simulink model "MovementMaker"  (R2021b)
settings: Solver=FixedStepAuto  StartTime=0.0  StopTime=10.0  FixedStep=.01  RelTol=1e-3
settings Model: Creator=Spino.shop  LastModifiedBy=Spino.shop

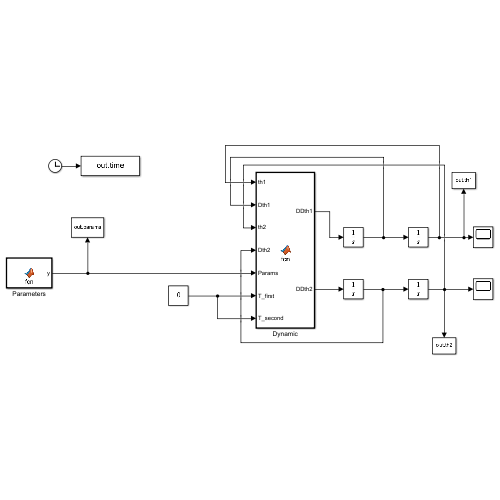
[thumbnail: Simulink's stored preview of the top-level diagram]
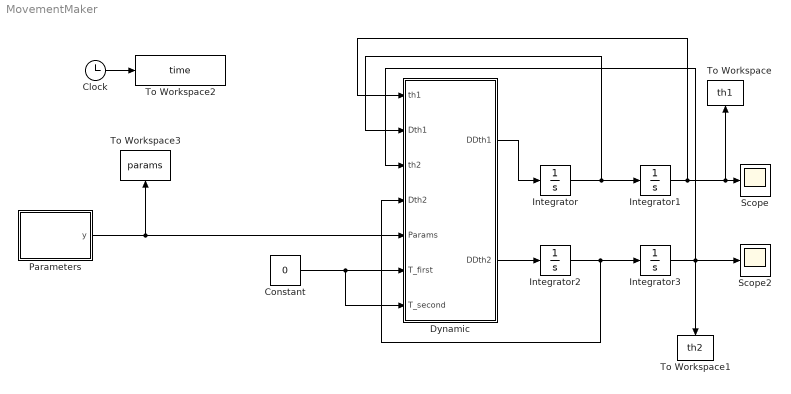
== system MovementMaker ==
  Clock : Clock
  Constant : Constant  Value=0
  Dynamic : MATLAB Function  TreatAsAtomicUnit=on
  Integrator{,1..3} (4 alike) : Integrator
  Parameters : MATLAB Function  TreatAsAtomicUnit=on
  Scope : Scope
  Scope2 : Scope
  To Workspace : ToWorkspace  VariableName=th1  SampleTime=-1
      settings: Save2DSignal=2-D array (concatenate along first dimension)
  To Workspace1 : ToWorkspace  VariableName=th2  SampleTime=-1
      settings: Save2DSignal=2-D array (concatenate along first dimension)
  To Workspace2 : ToWorkspace  VariableName=time  SampleTime=-1
      settings: Save2DSignal=2-D array (concatenate along first dimension)
  To Workspace3 : ToWorkspace  VariableName=params
      settings: MaxDataPoints=1  Save2DSignal=2-D array (concatenate along first dimension)
  wires:
  Integrator/1 -> Dynamic/2(Dth1), Integrator1/1
  Dynamic/1(DDth1) -> Integrator/1
  Parameters/1(y) -> To Workspace3/1, Dynamic/5(Params)
  Clock/1 -> To Workspace2/1
  Integrator2/1 -> Dynamic/4(Dth2), Integrator3/1
  Dynamic/2(DDth2) -> Integrator2/1
  Integrator1/1 -> Dynamic/1(th1), Scope/1, To Workspace/1
  Integrator3/1 -> Dynamic/3(th2), Scope2/1, To Workspace1/1
  Constant/1 -> Dynamic/6(T_first), Dynamic/7(T_second)

== matlab function MovementMaker/Dynamic ==
  data: th1 input; DDth1 output; Dth1 input; th2 input; Dth2 input; Params input; T_first input; T_second input; DDth2 output
function [DDth1,DDth2]  = fcn(th1, Dth1, th2, Dth2, Params, T_first, T_second)

    m1=Params(1); % First arm's mass (kg)
    m2 =Params(2); % Second arm's mass (kg)
    g =Params(3); % Gravity constant
    c1 =Params(4); % Damping coeff of first joint
    c2 =Params(5); % Damping coeff of second joint
    Kt1 =Params(6); % Spring coeff of first joint
    Kt2 =Params(7); % Spring coeff of second joint
    l1 =Params(8); % First arm's length (m)
    l2 =Params(9); % Second arm's length(m)
    lc1=Params(10); % Distance of center of mass of forearm from elbow joint(m)
    lc2 =Params(11); % Distance of center of mass of hand from wrist joint(m)

    T1 = T_first; 
    T2 = T_second;

    Y = zeros(4,1);
    Y(1) = th1;
    Y(2) = Dth1;
    Y(3) = th2;
    Y(4) = Dth2;


    
    DDth1 = -(Kt1*lc1^2*Y(1) - T1*lc1^2 + c1*lc1^2*Y(2) + cos(Y(1))*g*lc1^3*m1 + ...
        cos(Y(1) - Y(3))*T2*l1*lc2 - cos(Y(1) - Y(3))*Kt2*l1*lc2*Y(3) - ...
        cos(Y(1) - Y(3))*c2*l1*lc2*Y(4) + cos(Y(1))*g*l1*lc1^2*m2 + ...
        cos(Y(1) - Y(3))*sin(Y(1) - Y(3))*l1^2*lc2^2*m2*Y(2)^2 - cos(Y(3))*cos(Y(1) - ...
        Y(3))*g*l1*lc2^2*m2 + sin(Y(1) - Y(3))*l1*lc1^2*lc2*m2*Y(4)^2)/(- m2*cos(Y(1) - Y(3))^2*l1^2*lc2^2 + ...
        m2*l1^2*lc1^2 + m1*lc1^4);
    
    
    DDth2 = (T2*l1^2*m2 + T2*lc1^2*m1 - c2*l1^2*m2*Y(4) - c2*lc1^2*m1*Y(4) - ...
        Kt2*l1^2*m2*Y(3) - Kt2*lc1^2*m1*Y(3) - cos(Y(1) - Y(3))*T1*l1*lc2*m2 + ...
        sin(Y(1) - Y(3))*l1^3*lc2*m2^2*Y(2)^2 - cos(Y(3))*g*l1^2*lc2*m2^2 + ...
        cos(Y(1) - Y(3))*Kt1*l1*lc2*m2*Y(1) + cos(Y(1) - Y(3))*c1*l1*lc2*m2*Y(2) - ...
        cos(Y(3))*g*lc1^2*lc2*m1*m2 + cos(Y(1))*cos(Y(1) - Y(3))*g*l1^2*lc2*m2^2 + ...
        cos(Y(1) - Y(3))*sin(Y(1) - Y(3))*l1^2*lc2^2*m2^2*Y(4)^2 + ...
        sin(Y(1) - Y(3))*l1*lc1^2*lc2*m1*m2*Y(2)^2 + ...
        cos(Y(1))*cos(Y(1) - Y(3))*g*l1*lc1*lc2*m1*m2)/(m2*(- m2*cos(Y(1) - Y(3))^2*l1^2*lc2^2 + ...
        m2*l1^2*lc1^2 + m1*lc1^4));
    
end

== matlab function MovementMaker/Parameters ==
  data: y output
function y = fcn()
    m1=1.1826; % First arm's mass (kg)
    m2 =0.4453; % Second arm's mass (kg)
    g =9.81; % Gravity constant
    c1 =.01; % Damping coeff of first joint
    c2 =0; % Damping coeff of second joint
    Kt1 =0; % Spring coeff of first joint
    Kt2 =0; % Spring coeff of second joint
    l1 =0.2513; % First arm's length (m)
    l2 =0.1899; % Second arm's length(m)
    lc1=0.1166; % Distance of center of mass of forearm from elbow joint(m)
    lc2 =0.0701; % Distance of center of mass of hand from wrist joint(m)
    y = [m1 m2 g c1 c2 Kt1 Kt2 l1 l2 lc1 lc2 ];

end
